simulink model "lab2_sim"  (R2015a)
settings: Solver=ode45  StartTime=0.0  StopTime=10.0  RelTol=1e-3
values from neighbouring files (symbols this model uses):
  A = [1.37189711143 1 0 0 0 0 0.796247030428 0 1 0 0 0 ... (36 elements, 6x6)]    [matrizes.mat]
  B = [1 0 0 0 0 0]    [matrizes.mat]
  C = [0.176432501593 -0.307260665336 -0.097075632123 0.119078500307 -0.365349527089 0]    [matrizes.mat]
  D = 0    [matrizes.mat]
  K = [0.152892335406 -0.0494306399458 -0.17992491845 0.0741519455973 0.109452261993 -0.0633139239932]    [matrizes.mat]
  M = [-4.02099236255 -3.77131879733 -2.84355374965 -1.32107837653 -1.17257932747 0.607476554194]    [matrizes.mat]
  Nbar = -2.20135488168    [matrizes.mat]    (also in script_lab2.m = Nu+K*Nx)
settings Model: Creator=Alunos  LastModifiedBy=Alunos

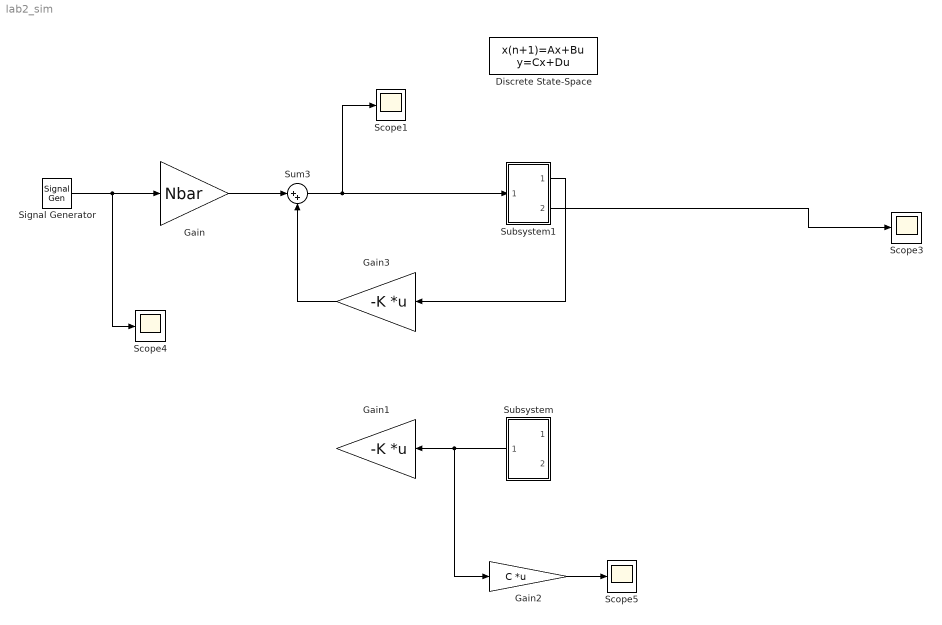
== system lab2_sim ==
  Discrete State-Space : DiscreteStateSpace  A=A  B=B  C=C  D=D  SampleTime=0.02
  Gain : Gain  Gain=Nbar
  Gain1 : Gain  Gain=-K  Multiplication=Matrix(K*u) (u vector)
  Gain2 : Gain  Gain=C  Multiplication=Matrix(K*u) (u vector)
  Gain3 : Gain  Gain=-K  Multiplication=Matrix(K*u) (u vector)
  Scope{1,3..5} (4 alike) : Scope
      Scope1 settings: SaveName=y_simulado3
      Scope3 settings: SaveName=y_simulado
      Scope4 settings: SaveName=y_simulado1
      Scope5 settings: SaveName=y_simulado2
  Signal Generator : SignalGenerator  WaveForm=square  Amplitude=43  Frequency=0.2
  Subsystem : Subsystem
  Subsystem1 : Subsystem
  Sum3 : Sum  Inputs=|++
  wires:
  Subsystem/1(Out1) -> Gain2/1, Gain1/1
  Signal Generator/1 -> Scope4/1, Gain/1
  Gain2/1 -> Scope5/1
  Sum3/1 -> Scope1/1, Subsystem1/1(In1)
  Gain/1 -> Sum3/1
  Subsystem1/2(Out2) -> Scope3/1
  Gain3/1 -> Sum3/2
  Subsystem1/1(Out1) -> Gain3/1

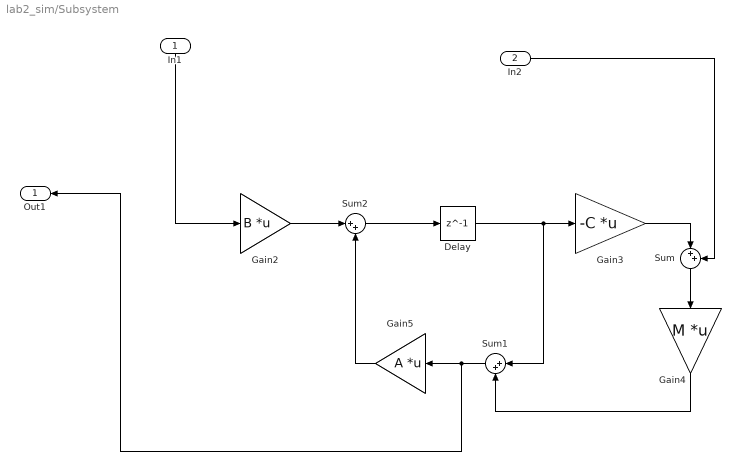
== system lab2_sim/Subsystem ==
  In1 : Inport
  In2 : Inport  Port=2
  Delay : Delay  DelayLength=1  InitialCondition=0  SampleTime=0.02
  Gain2 : Gain  Gain=B  Multiplication=Matrix(K*u) (u vector)
  Gain3 : Gain  Gain=-C  Multiplication=Matrix(K*u) (u vector)
  Gain4 : Gain  Gain=M  Multiplication=Matrix(K*u) (u vector)
  Gain5 : Gain  Gain=A  Multiplication=Matrix(K*u) (u vector)
  Sum : Sum  Inputs=|++
  Sum1 : Sum  Inputs=|++
  Sum2 : Sum  Inputs=|++
  Out1 : Outport
  wires:
  Gain3/1 -> Sum/1
  In1/1 -> Gain2/1
  Gain4/1 -> Sum1/2
  Sum/1 -> Gain4/1
  Gain5/1 -> Sum2/2
  Sum1/1 -> Out1/1, Gain5/1
  In2/1 -> Sum/2
  Sum2/1 -> Delay/1
  Delay/1 -> Sum1/1, Gain3/1
  Gain2/1 -> Sum2/1

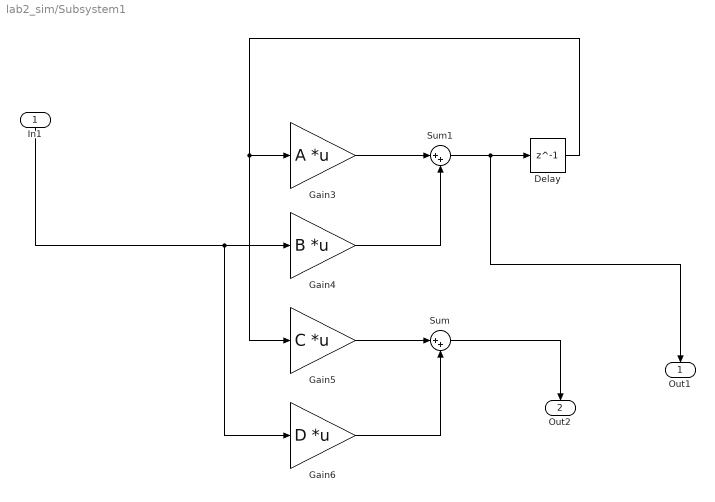
== system lab2_sim/Subsystem1 ==
  In1 : Inport
  Delay : Delay  DelayLength=1  InitialCondition=0  SampleTime=0.02
  Gain3 : Gain  Gain=A  Multiplication=Matrix(K*u) (u vector)
  Gain4 : Gain  Gain=B  Multiplication=Matrix(K*u) (u vector)
  Gain5 : Gain  Gain=C  Multiplication=Matrix(K*u) (u vector)
  Gain6 : Gain  Gain=D  Multiplication=Matrix(K*u) (u vector)
  Sum : Sum  Inputs=|++
  Sum1 : Sum  Inputs=|++
  Out1 : Outport
  Out2 : Outport  Port=2
  wires:
  Gain4/1 -> Sum1/2
  Delay/1 -> Gain5/1, Gain3/1
  In1/1 -> Gain6/1, Gain4/1
  Sum1/1 -> Out1/1, Delay/1
  Gain5/1 -> Sum/1
  Gain6/1 -> Sum/2
  Gain3/1 -> Sum1/1
  Sum/1 -> Out2/1
